simulink model "Jakub_Bączyk_1_Projekt_2_Ukl_o"  (R2015a)
settings: Solver=ode45  StartTime=0.0  StopTime=50  FixedStep=0.001  RelTol=1e-3
undefined symbols (not defined in the file): b1
settings Model: Creator=238  LastModifiedBy=lenovo

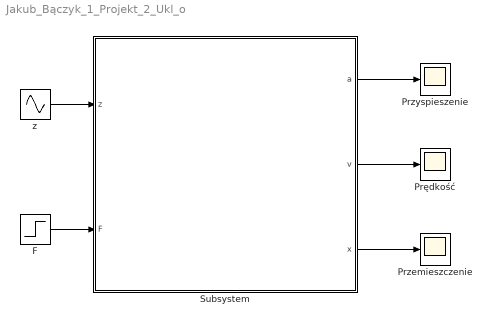
== system Jakub_Bączyk_1_Projekt_2_Ukl_o ==
  F : Step  Time=0  SampleTime=0
  Przemieszczenie : Scope
  Przyspieszenie : Scope
  Prędkość : Scope
      settings: SaveName=ScopeData2
  Subsystem : Subsystem  mask(Układ masa sprężyna tłumik){m=0, v0=0, x0=0, c1=0, c2=0, bb1=1, b2=0}
      mask prompts: m "Masa [kg]"; v0 "Prędkość początkowa [m/s]"; x0 "Przemieszczenie początkowe [m/s]"; c1 "Sztywnosc sprezyny c1[]"; c2 "Sztywnosc sprezyny c2[]"; bb1 "Wspolczynnik tlumienia b1[]"; b2 "Wspolczynnik tlumienia b2[]"
      mask help:
      | Zmodelowany układ mechaniczny, który opiera się na 2 tłumikach b1 oraz 2
      | tłumikach b2 i sprężynach oraz c2. Na klocek działają wymuszenie siłowe (F) oraz kinematyczne (z).
      | Przemieszczenie zostało określone jako "x". Poniżej można wprowadzić
      | parametry pozwalające śledzić charakterystykę zachowania się układu.
      mask Help:
      | <html>
      | <img src="E:\studia Albert\programy użytkowe\projekt 2\schemat a.png">
      | Równanie różniczkowe opisującego tego typu układy:
      | <img src="E:\studia Albert\programy użytkowe\projekt 2\równanie.png">
      | <p> Sygnały wejściowe modelu to:
      | F- wymuszenie siłowe
      | z- wymuszenie kinematyczne
      | </p>
      | <p> Parametry układu:
      | m- masa klocka
      | v0-prędkość początkowa klocka
      | x0-przemieszczenie początkowe klocka
      | b1,b2,b3- wartość tłumienia poszczególnych tłumików
      | c1,c2,c3- wartość sztywności poszczególnych sprężyn
      | </p>
      | <p> Przebiegi, które możemy rejestrować:
      | x- przemieszczenie się klocka
      | v- prędkość klocka
      | a- przyspieszenie klocka
      | </p>
      | Aby zobaczyć przebieg charakterystyki należy kliknąć na odpowiedni wyświetlacz.
      | <p>
      | Uwagi!
      | - wpisywana masa musi być dodatnia
      | -należy podać wszystkie parametry w celu odzwierciedlenia przebiegu
      | </html>
      mask Callback m:
      | if str2num(get_param(gcb,'m'))<=0
      |     error('masa musi być dodatnia')
      | end
      mask TypeOptions bb1: 1 | 2 | 3 | 4 | 5 | 6 | 7 | 8 | 9 | 10
      mask Callback bb1: b1=str2num(get_param(gcb,'bb1'));
      mask Display:
      | color('blue') %kolor lini
      | %kreski pod linią
      | plot([0.12 0.09],[0.1 0.05])
      | plot([0.15 0.12],[0.1 0.05])
      | plot([0.18 0.15],[0.1 0.05])
      | plot([0.21 0.18],[0.1 0.05])
      | plot([0.24 0.21],[0.1 0.05])
      | plot([0.27 0.24],[0.1 0.05])
      | plot([0.30 0.27],[0.1 0.05])
      | plot([0.33 0.3],[0.1 0.05])
      | plot([0.36 0.33],[0.1 0.05])
      | plot([0.39 0.36],[0.1 0.05])
      | plot([0.42 0.39],[0.1 0.05])
      | plot([0.45 0.42,],[0.1 0.05])
      | plot([0.48 0.45],[0.1 0.05])
      | plot([0.51 0.48],[0.1 0.05])
      | plot([0.54 0.51],[0.1 0.05])
      | plot([0.57 0.54],[0.1 0.05])
      | plot([0.6 0.57],[0.1 0.05])
      | plot([0.63 0.6],[0.1 0.05])
      | plot([0.66 0.63],[0.1 0.05])
      | plot([0.69 0.66],[0.1 0.05])
      | plot([0.72 0.69],[0.1 0.05])
      | plot([0.75 0.72],[0.1 0.05])
      | plot([0.78 0.75],[0.1 0.05])
      | plot([0.81 0.78],[0.1 0.05])
      | plot([0.84 0.81],[0.1 0.05])
      | plot([0.87 0.84],[0.1 0.05])
      | plot([0.1 0.9],[0.1 0.1])%współrzędne x i y, pierwsza linia pozioma
      | plot([0.1 0.9],[0.105 0.105])%pogrubienie linii
      | plot([0.1 0.9],[0.103 0.103]) %pogrubienie linii
      | %tłumik b2 dolny
      | plot([0.33 0.33],[0.1 0.15]) %pod tłumikem
      | plot([0.28 0.38],[0.15 0.15])
      | plot([0.28 0.28],[0.15 0.18])
      | plot([0.38 0.38],[0.15 0.18])
      | plot([0.29 0.37],[0.18 0.18])
      | plot([0.33 0.33],[0.18 0.21]) %nad tłumikiem
      | %tłumik b1 dolny
      | plot([0.5 0.5],[0.1 0.15]) %pod tłumikem
      | plot([0.45 0.55],[0.15 0.15])
      | plot([0.45 0.45],[0.15 0.18])
      | plot([0.55 0.55],[0.15 0.18])
      | plot([0.46 0.54],[0.18 0.18])
      | plot([0.5 0.5],[0.18 0.21]) %nad tłumikiem
      | plot([0.33 0.5],[0.21 0.21]) %połączenie
      | plot([0.415 0.415],[0.21 0.23]) %kreska nad
      | plot([0.33 0.5],[0.23 0.23]) %połączenie
      | %tłumik b2 górny
      | plot([0.33 0.33],[0.23 0.26])%pod tłumikiem
      | plot([0.28 0.38],[0.26 0.26])
      | plot([0.28 0.28],[0.26 0.29])
      | plot([0.38 0.38],[0.26 0.29])
      | plot([0.29 0.37],[0.29 0.29])
      | plot([0.33 0.33],[0.29 0.32])%nad tłumikiem
      | %tłumik b1 górny
      | plot([0.5 0.5],[0.23 0.26]) %pod tłumikem
      | plot([0.45 0.55],[0.26 0.26])
      | plot([0.45 0.45],[0.26 0.29])
      | plot([0.55 0.55],[0.26 0.29])
      | plot([0.46 0.54],[0.29 0.29])
      | plot([0.5 0.5],[0.29 0.32]) %nad tłumikiem
      | plot([0.33 0.5],[0.32 0.32]) %połączenie
      | plot([0.415 0.415],[0.32 0.38]) %kreska nad
      | %sprężyna c2
      | plot([0.7 0.7],[0.1 0.15]) %pod spręzyną
      | plot([0.7 0.65],[0.15 0.16])
      | plot([0.65 0.75],[0.16 0.17])
      | plot([0.75 0.65],[0.17 0.185])
      | plot([0.75 0.65],[0.17 0.185])
      | plot([0.65 0.75],[0.185 0.2])
      | plot([0.75 0.7],[0.2 0.21])
      | plot([0.7 0.7],[0.21 0.27]) %nad sprężyną c2
      | %sprężyna c2
      | plot([0.7 0.65],[0.27 0.28])
      | plot([0.65 0.75],[0.28 0.29])
      | plot([0.75 0.65],[0.29 0.305])
      | plot([0.75 0.65],[0.29 0.305])
      | plot([0.65 0.75],[0.305 0.32])
      | plot([0.75 0.7],[0.32 0.33])
      | plot([0.7 0.7],[0.33 0.38])%nad sprężyną c1
      | %masa
      | plot([0.3 0.8],[0.38 0.38])
      | plot([0.3 0.8],[0.68 0.68])
      | plot([0.3 0.3],[0.38 0.68])
      | plot([0.8 0.8],[0.38 0.68])
      | %strzałka dla x
      | plot([0.3 0.15],[0.6 0.6])
      | plot([0.18 0.18],[0.6 0.52])
      | %strzałka dla z
      | plot([0.445 0.445],[0.8 0.68])
      | %strzałka dla F
      | plot([0.65 0.65],[0.8 0.68])
      | patch([0.178 0.189 0.2],[0.53 0.495 0.53],[0 0 1])%grot dla x
      | patch([0.43 0.45 0.47],[0.71 0.675 0.71],[0 0 1])%grot dla z
      | patch([0.63 0.65 0.67],[0.71 0.675 0.71],[0 0 1])%grot dla F
      | color('black')
      | %opis parametrów
      | text(0.55,0.55,'m')
      | text(0.22,0.2,'b2')
      | text(0.22,0.3,'b2')
      | text(0.58,0.2,'b1')
      | text(0.58,0.3,'b1')
      | text(0.75,0.23,'c2')
      | text(0.75,0.35,'c1')
      | text(0.21,0.55,'x')
      | text(0.45,0.85,'z')
      | text(0.65,0.85,'F')
      | %opis wejść/wyjść
      | port_label('output', 1, 'a')
      | port_label('output', 2, 'v')
      | port_label('output', 3, 'x')
      | port_label('input', 1, 'z')
      | port_label('input', 2, 'F')
  z : Sin  Amplitude=0  Frequency=0  SampleTime=0
  wires:
  z/1 -> Subsystem/1(z)
  F/1 -> Subsystem/2(F)
  Subsystem/1(a) -> Przyspieszenie/1
  Subsystem/2(v) -> Prędkość/1
  Subsystem/3(x) -> Przemieszczenie/1

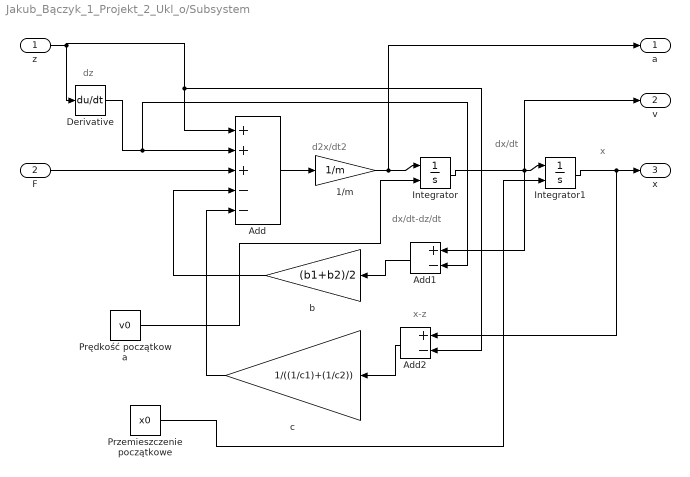
== system Jakub_Bączyk_1_Projekt_2_Ukl_o/Subsystem ==
  note: dz
  note: x-z
  note: dx/dt-dz/dt
  note: x
  note: dx/dt
  note: d2x/dt2
  z : Inport
  F : Inport  Port=2
  1/m : Gain  Gain=1/m
  Add : Sum  Inputs=+++--
  Add1 : Sum  Inputs=+-
  Add2 : Sum  Inputs=+-
  Derivative : Derivative
  Integrator : Integrator  InitialConditionSource=external
  Integrator1 : Integrator  InitialConditionSource=external
  Przemieszczenie początkowe : Constant  Value=x0
  Prędkość początkowa : Constant  Value=v0
  b : Gain  Gain=(b1+b2)/2
  c : Gain  Gain=1/((1/c1)+(1/c2))
  a : Outport
  v : Outport  Port=2
  x : Outport  Port=3
  wires:
  c/1 -> Add/5
  Integrator1/1 -> x/1, Add2/1
  F/1 -> Add/3
  Integrator/1 -> v/1, Add1/1, Integrator1/1
  1/m/1 -> a/1, Integrator/1
  Add2/1 -> c/1
  Add1/1 -> b/1
  Derivative/1 -> Add1/2, Add/2
  z/1 -> Add2/2, Add/1, Derivative/1
  Add/1 -> 1/m/1
  b/1 -> Add/4
  Prędkość początkowa/1 -> Integrator/2
  Przemieszczenie początkowe/1 -> Integrator1/2
